simulink model "SMA_Wire_Sim"  (R2023b)
settings: Solver=VariableStepAuto  StartTime=0.0  StopTime=10  RelTol=1e-5
values from neighbouring files (symbols this model uses):
  Da = 75.0e9    (= 75000000000)    [Initialization.m]
  dens = 6450.0    (= 6450)    [Initialization.m]
  Dm = 28.0e9    (= 28000000000)    [Initialization.m]
  Dw = 0.00031    [Initialization.m]
  epsR = 0.05    [Initialization.m]
  epsR1 = 0.036    [Initialization.m]
  Length = 0.18    [Initialization.m]
  Lw1 = 0.18    [Initialization.m]
  Lw2 = 0.18    [Initialization.m]
  pa = 100*10^-8    (= 1e-06)    [Initialization.m]
  pm = 80*10^-8    (= 8e-07)    [Initialization.m]
  SectA = pi*(Diameter^2)/4    (= 7.54767635025e-08)    [Initialization.m]
  sigma0 = (disp_i*Ks)/SectA    (= 2649822.15346)    [Initialization.m]
  Tamb = 25    [Initialization.m]
  thetaT = 0    [Initialization.m]
libraries: nesl_utility x10, ee_lib x10, fl_lib x8, simulink_extras x4, simulink x3
(part 2 of 2)

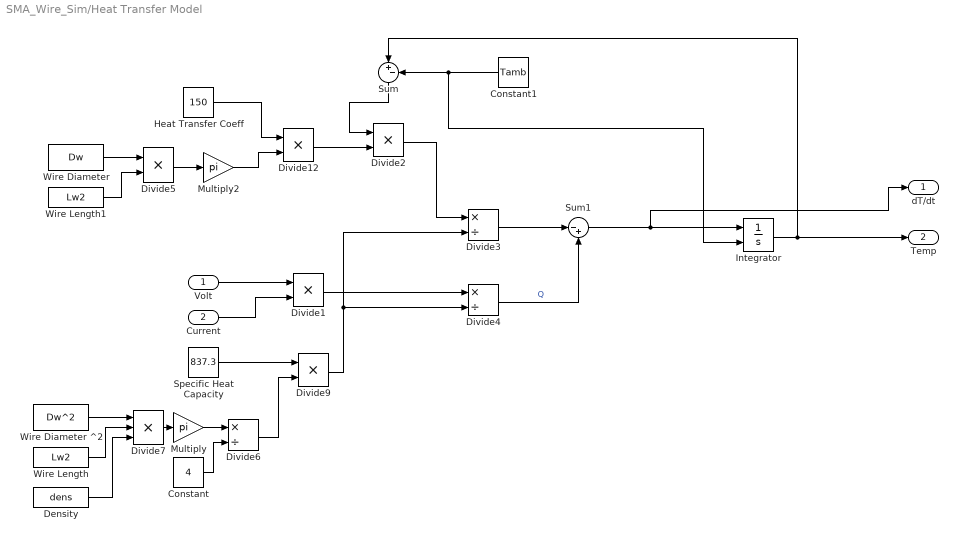
== system SMA_Wire_Sim/Heat Transfer Model ==
  Volt : Inport
  Current : Inport  Port=2
  Constant : Constant  Value=4
  Constant1 : Constant  Value=Tamb
  Density : Constant  Value=dens
  Divide{1..2,5,9,12} (5 alike) : Product  Inputs=**
  Divide3 : Product  Inputs=*/
  Divide4 : Product  Inputs=*/
  Divide6 : Product  Inputs=*/
  Divide7 : Product  Inputs=***
  Heat Transfer Coeff : Constant  Value=150
  Integrator : Integrator  InitialConditionSource=external  InitialCondition=25
  Multiply : Gain  Gain=pi
  Multiply2 : Gain  Gain=pi
  Specific Heat Capacity : Constant  Value=837.3
  Sum : Sum  Inputs=|+-
  Sum1 : Sum  Inputs=|-+
  Wire Diameter : Constant  Value=Dw
  Wire Diameter ^2 : Constant  Value=Dw^2
  Wire Length : Constant  Value=Lw2
  Wire Length1 : Constant  Value=Lw2
  dT/dt : Outport
  Temp : Outport  Port=2
  wires:
  Current/1 -> Divide1/2
  Volt/1 -> Divide1/1
  Constant1/1 -> Integrator/2, Sum/2
  Divide1/1 -> Divide4/1
  Wire Diameter ^2/1 -> Divide7/1
  Wire Length/1 -> Divide7/2
  Divide7/1 -> Multiply/1
  Divide3/1 -> Sum1/1
  Sum1/1 -> dT/dt/1, Integrator/1
  Divide4/1 -> Sum1/2  "Q"
  Density/1 -> Divide7/3
  Specific Heat Capacity/1 -> Divide9/1
  Multiply/1 -> Divide6/1
  Constant/1 -> Divide6/2
  Divide9/1 -> Divide3/2, Divide4/2
  Divide6/1 -> Divide9/2
  Sum/1 -> Divide2/1
  Divide2/1 -> Divide3/1
  Divide5/1 -> Multiply2/1
  Wire Length1/1 -> Divide5/2
  Wire Diameter/1 -> Divide5/1
  Multiply2/1 -> Divide12/2
  Heat Transfer Coeff/1 -> Divide12/1
  Divide12/1 -> Divide2/2
  Integrator/1 -> Sum/1, Temp/1

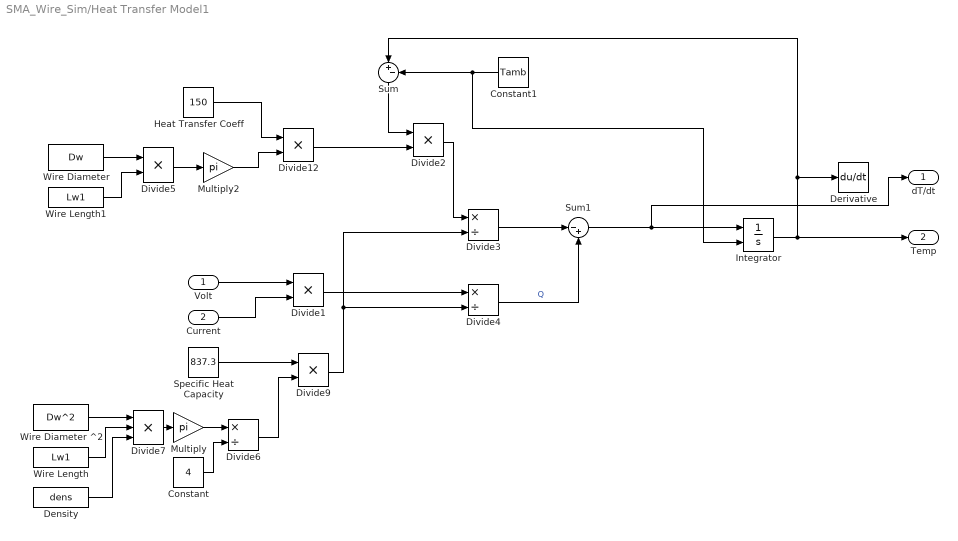
== system SMA_Wire_Sim/Heat Transfer Model1 ==
  Volt : Inport
  Current : Inport  Port=2
  Constant : Constant  Value=4
  Constant1 : Constant  Value=Tamb
  Density : Constant  Value=dens
  Derivative : Derivative
  Divide{1..2,5,9,12} (5 alike) : Product  Inputs=**
  Divide3 : Product  Inputs=*/
  Divide4 : Product  Inputs=*/
  Divide6 : Product  Inputs=*/
  Divide7 : Product  Inputs=***
  Heat Transfer Coeff : Constant  Value=150
  Integrator : Integrator  InitialConditionSource=external  InitialCondition=25
  Multiply : Gain  Gain=pi
  Multiply2 : Gain  Gain=pi
  Specific Heat Capacity : Constant  Value=837.3
  Sum : Sum  Inputs=|+-
  Sum1 : Sum  Inputs=|-+
  Wire Diameter : Constant  Value=Dw
  Wire Diameter ^2 : Constant  Value=Dw^2
  Wire Length : Constant  Value=Lw1
  Wire Length1 : Constant  Value=Lw1
  dT/dt : Outport
  Temp : Outport  Port=2
  wires:
  Current/1 -> Divide1/2
  Volt/1 -> Divide1/1
  Constant1/1 -> Sum/2, Integrator/2
  Divide1/1 -> Divide4/1
  Wire Diameter ^2/1 -> Divide7/1
  Wire Length/1 -> Divide7/2
  Divide7/1 -> Multiply/1
  Divide3/1 -> Sum1/1
  Sum1/1 -> dT/dt/1, Integrator/1
  Divide4/1 -> Sum1/2  "Q"
  Density/1 -> Divide7/3
  Specific Heat Capacity/1 -> Divide9/1
  Multiply/1 -> Divide6/1
  Constant/1 -> Divide6/2
  Divide9/1 -> Divide3/2, Divide4/2
  Divide6/1 -> Divide9/2
  Sum/1 -> Divide2/1
  Divide2/1 -> Divide3/1
  Divide5/1 -> Multiply2/1
  Wire Length1/1 -> Divide5/2
  Wire Diameter/1 -> Divide5/1
  Multiply2/1 -> Divide12/2
  Heat Transfer Coeff/1 -> Divide12/1
  Divide12/1 -> Divide2/2
  Integrator/1 -> Derivative/1, Sum/1, Temp/1

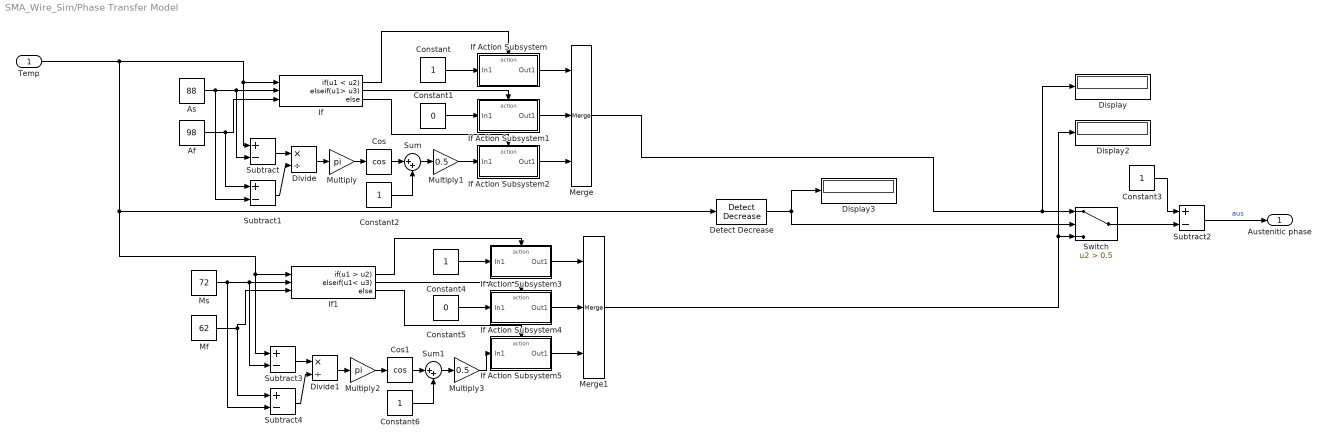
== system SMA_Wire_Sim/Phase Transfer Model ==
  Temp : Inport
  Af : Constant  Value=98
  As : Constant  Value=88
  Constant{,2..4,6} (5 alike) : Constant
  Constant1 : Constant  Value=0
  Constant5 : Constant  Value=0
  Cos : Trigonometry  Operator=cos
  Cos1 : Trigonometry  Operator=cos
  Detect Decrease : simulink/Logic and Bit Operations/Detect Decrease  vinit=0  OutDataTypeStr=uint8
  Display : Display
  Display2 : Display
  Display3 : Display
  Divide : Product  Inputs=*/
  Divide1 : Product  Inputs=*/
  If : If  NumInputs=3  IfExpression=u1 < u2  ElseIfExpressions=u1> u3
  If Action Subsystem : Subsystem  TreatAsAtomicUnit=on
  If Action Subsystem1 : Subsystem  TreatAsAtomicUnit=on
  If Action Subsystem2 : Subsystem  TreatAsAtomicUnit=on
  If Action Subsystem3 : Subsystem  TreatAsAtomicUnit=on
  If Action Subsystem4 : Subsystem  TreatAsAtomicUnit=on
  If Action Subsystem5 : Subsystem  TreatAsAtomicUnit=on
  If1 : If  NumInputs=3  IfExpression=u1 > u2  ElseIfExpressions=u1< u3
  Merge : Merge  Inputs=3
  Merge1 : Merge  Inputs=3
  Mf : Constant  Value=62
  Ms : Constant  Value=72
  Multiply : Gain  Gain=pi
  Multiply1 : Gain  Gain=0.5
  Multiply2 : Gain  Gain=pi
  Multiply3 : Gain  Gain=0.5
  Subtract{,1..4} (5 alike) : Sum  Inputs=+-
  Sum : Sum  Inputs=|++
  Sum1 : Sum  Inputs=|++
  Switch : Switch  Criteria=u2 > Threshold  Threshold=0.5  SaturateOnIntegerOverflow=off  InputSameDT=off
  "Austenitic phase " : Outport
  wires:
  As/1 -> Subtract1/2, Subtract/2, If/2
  Af/1 -> Subtract1/1, If/3
  If/1 -> If Action Subsystem/Action
  If/2 -> If Action Subsystem1/Action
  Constant/1 -> If Action Subsystem/1(In1)
  Constant1/1 -> If Action Subsystem1/1(In1)
  If/3 -> If Action Subsystem2/Action
  If Action Subsystem/1(Out1) -> Merge/1
  If Action Subsystem1/1(Out1) -> Merge/2
  If Action Subsystem2/1(Out1) -> Merge/3
  Subtract/1 -> Divide/1
  Subtract1/1 -> Divide/2
  Divide/1 -> Multiply/1
  Multiply/1 -> Cos/1
  Cos/1 -> Sum/1
  Constant2/1 -> Sum/2
  Sum/1 -> Multiply1/1
  Multiply1/1 -> If Action Subsystem2/1(In1)
  Constant3/1 -> Subtract2/1
  Divide1/1 -> Multiply2/1
  If Action Subsystem4/1(Out1) -> Merge1/2
  Multiply2/1 -> Cos1/1
  Mf/1 -> If1/3, Subtract4/1
  Cos1/1 -> Sum1/1
  Subtract3/1 -> Divide1/1
  Subtract4/1 -> Divide1/2
  Sum1/1 -> Multiply3/1
  Constant4/1 -> If Action Subsystem3/1(In1)
  If1/1 -> If Action Subsystem3/Action
  If1/3 -> If Action Subsystem5/Action
  If1/2 -> If Action Subsystem4/Action
  Constant5/1 -> If Action Subsystem4/1(In1)
  Ms/1 -> Subtract4/2, Subtract3/2, If1/2
  Constant6/1 -> Sum1/2
  Multiply3/1 -> If Action Subsystem5/1(In1)
  If Action Subsystem5/1(Out1) -> Merge1/3
  If Action Subsystem3/1(Out1) -> Merge1/1
  Temp/1 -> Detect Decrease/1, Subtract3/1, If1/1, Subtract/1, If/1
  Detect Decrease/1 -> Switch/2, Display3/1
  Merge1/1 -> Display2/1, Switch/3
  Merge/1 -> Display/1, Switch/1
  Switch/1 -> Subtract2/2
  Subtract2/1 -> "Austenitic phase "/1  "aus"

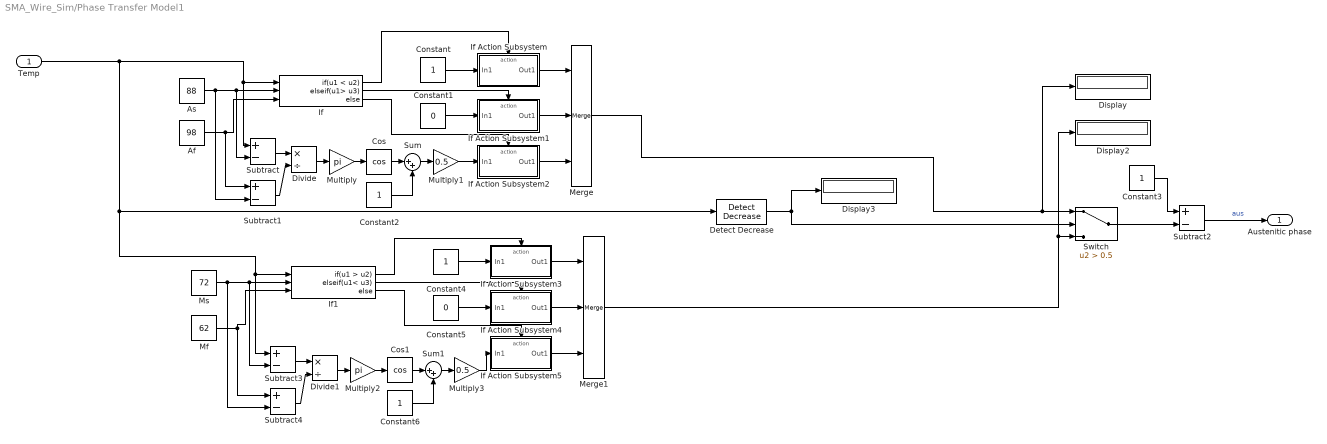
== system SMA_Wire_Sim/Phase Transfer Model1 ==
  Temp : Inport
  Af : Constant  Value=98
  As : Constant  Value=88
  Constant{,2..4,6} (5 alike) : Constant
  Constant1 : Constant  Value=0
  Constant5 : Constant  Value=0
  Cos : Trigonometry  Operator=cos
  Cos1 : Trigonometry  Operator=cos
  Detect Decrease : simulink/Logic and Bit Operations/Detect Decrease  vinit=0  OutDataTypeStr=uint8
  Display : Display
  Display2 : Display
  Display3 : Display
  Divide : Product  Inputs=*/
  Divide1 : Product  Inputs=*/
  If : If  NumInputs=3  IfExpression=u1 < u2  ElseIfExpressions=u1> u3
  If Action Subsystem : Subsystem  TreatAsAtomicUnit=on
  If Action Subsystem1 : Subsystem  TreatAsAtomicUnit=on
  If Action Subsystem2 : Subsystem  TreatAsAtomicUnit=on
  If Action Subsystem3 : Subsystem  TreatAsAtomicUnit=on
  If Action Subsystem4 : Subsystem  TreatAsAtomicUnit=on
  If Action Subsystem5 : Subsystem  TreatAsAtomicUnit=on
  If1 : If  NumInputs=3  IfExpression=u1 > u2  ElseIfExpressions=u1< u3
  Merge : Merge  Inputs=3
  Merge1 : Merge  Inputs=3
  Mf : Constant  Value=62
  Ms : Constant  Value=72
  Multiply : Gain  Gain=pi
  Multiply1 : Gain  Gain=0.5
  Multiply2 : Gain  Gain=pi
  Multiply3 : Gain  Gain=0.5
  Subtract{,1..4} (5 alike) : Sum  Inputs=+-
  Sum : Sum  Inputs=|++
  Sum1 : Sum  Inputs=|++
  Switch : Switch  Criteria=u2 > Threshold  Threshold=0.5  SaturateOnIntegerOverflow=off  InputSameDT=off
  "Austenitic phase " : Outport
  wires:
  As/1 -> Subtract1/2, Subtract/2, If/2
  Af/1 -> Subtract1/1, If/3
  If/1 -> If Action Subsystem/Action
  If/2 -> If Action Subsystem1/Action
  Constant/1 -> If Action Subsystem/1(In1)
  Constant1/1 -> If Action Subsystem1/1(In1)
  If/3 -> If Action Subsystem2/Action
  If Action Subsystem/1(Out1) -> Merge/1
  If Action Subsystem1/1(Out1) -> Merge/2
  If Action Subsystem2/1(Out1) -> Merge/3
  Subtract/1 -> Divide/1
  Subtract1/1 -> Divide/2
  Divide/1 -> Multiply/1
  Multiply/1 -> Cos/1
  Cos/1 -> Sum/1
  Constant2/1 -> Sum/2
  Sum/1 -> Multiply1/1
  Multiply1/1 -> If Action Subsystem2/1(In1)
  Constant3/1 -> Subtract2/1
  Divide1/1 -> Multiply2/1
  If Action Subsystem4/1(Out1) -> Merge1/2
  Multiply2/1 -> Cos1/1
  Mf/1 -> If1/3, Subtract4/1
  Cos1/1 -> Sum1/1
  Subtract3/1 -> Divide1/1
  Subtract4/1 -> Divide1/2
  Sum1/1 -> Multiply3/1
  Constant4/1 -> If Action Subsystem3/1(In1)
  If1/1 -> If Action Subsystem3/Action
  If1/3 -> If Action Subsystem5/Action
  If1/2 -> If Action Subsystem4/Action
  Constant5/1 -> If Action Subsystem4/1(In1)
  Ms/1 -> Subtract4/2, Subtract3/2, If1/2
  Constant6/1 -> Sum1/2
  Multiply3/1 -> If Action Subsystem5/1(In1)
  If Action Subsystem5/1(Out1) -> Merge1/3
  If Action Subsystem3/1(Out1) -> Merge1/1
  Temp/1 -> Detect Decrease/1, Subtract3/1, If1/1, Subtract/1, If/1
  Detect Decrease/1 -> Switch/2, Display3/1
  Merge1/1 -> Display2/1, Switch/3
  Merge/1 -> Display/1, Switch/1
  Switch/1 -> Subtract2/2
  Subtract2/1 -> "Austenitic phase "/1  "aus"

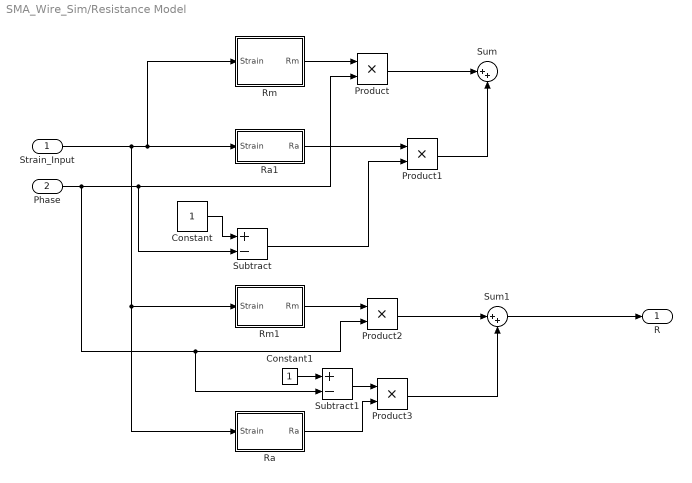
== system SMA_Wire_Sim/Resistance Model ==
  Strain_Input : Inport
  Phase : Inport  Port=2
  Constant : Constant
  Constant1 : Constant
  Product{,1..3} (4 alike) : Product
  Ra : Subsystem
  Ra1 : Subsystem
  Rm : Subsystem
  Rm1 : Subsystem
  Subtract : Sum  Inputs=+-
  Subtract1 : Sum  Inputs=+-
  Sum : Sum  Inputs=|++
  Sum1 : Sum  Inputs=|++
  R : Outport
  wires:
  Rm/1(Rm) -> Product/1
  Product/1 -> Sum/1
  Constant/1 -> Subtract/1
  Ra1/1(Ra) -> Product1/1
  Subtract/1 -> Product1/2
  Product1/1 -> Sum/2
  Strain_Input/1 -> Ra/1(Strain), Rm1/1(Strain), Ra1/1(Strain), Rm/1(Strain)
  Product3/1 -> Sum1/2
  Constant1/1 -> Subtract1/1
  Rm1/1(Rm) -> Product2/1
  Subtract1/1 -> Product3/1
  Product2/1 -> Sum1/1
  Ra/1(Ra) -> Product3/2
  Phase/1 -> Subtract1/2, Product2/2, Product/2, Subtract/2
  Sum1/1 -> R/1

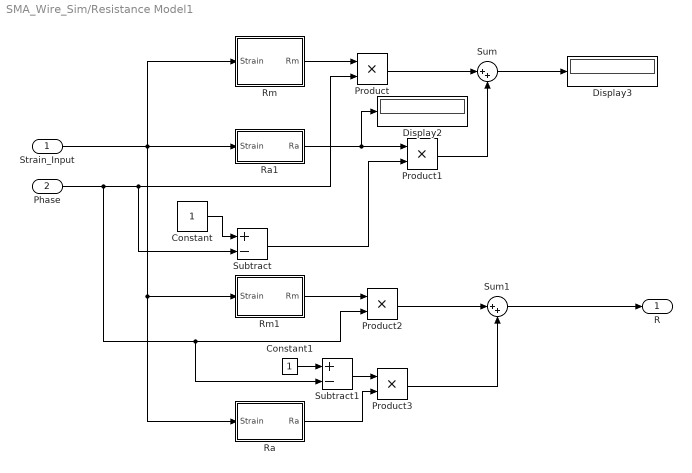
== system SMA_Wire_Sim/Resistance Model1 ==
  Strain_Input : Inport
  Phase : Inport  Port=2
  Constant : Constant
  Constant1 : Constant
  Display2 : Display
  Display3 : Display
  Product{,1..3} (4 alike) : Product
  Ra : Subsystem
  Ra1 : Subsystem
  Rm : Subsystem
  Rm1 : Subsystem
  Subtract : Sum  Inputs=+-
  Subtract1 : Sum  Inputs=+-
  Sum : Sum  Inputs=|++
  Sum1 : Sum  Inputs=|++
  R : Outport
  wires:
  Rm/1(Rm) -> Product/1
  Product/1 -> Sum/1
  Constant/1 -> Subtract/1
  Ra1/1(Ra) -> Display2/1, Product1/1
  Subtract/1 -> Product1/2
  Product1/1 -> Sum/2
  Sum/1 -> Display3/1
  Strain_Input/1 -> Rm/1(Strain), Ra/1(Strain), Rm1/1(Strain), Ra1/1(Strain)
  Product3/1 -> Sum1/2
  Constant1/1 -> Subtract1/1
  Rm1/1(Rm) -> Product2/1
  Subtract1/1 -> Product3/1
  Product2/1 -> Sum1/1
  Ra/1(Ra) -> Product3/2
  Phase/1 -> Subtract1/2, Product2/2, Product/2, Subtract/2
  Sum1/1 -> R/1

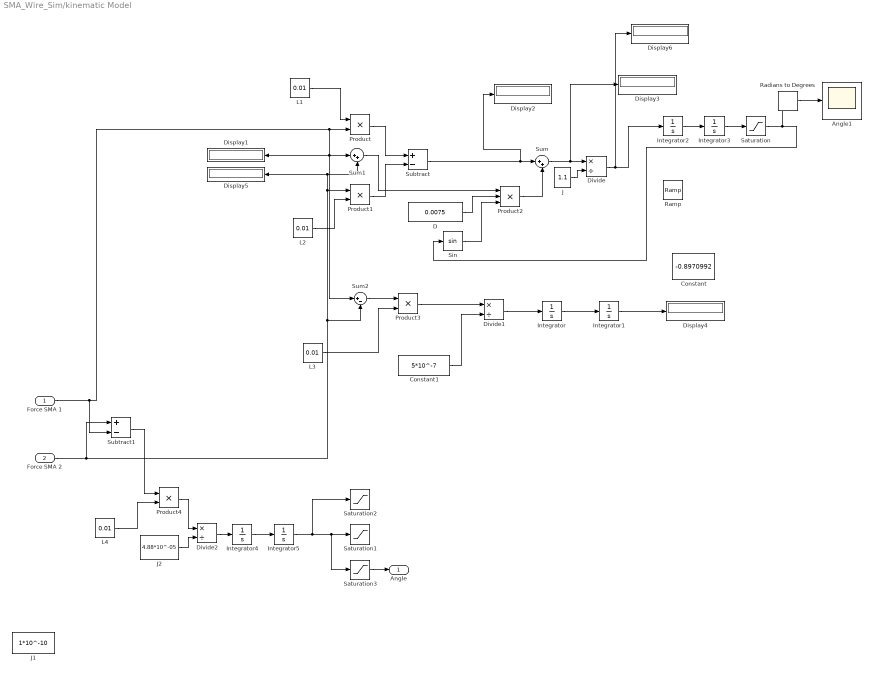
== system SMA_Wire_Sim/kinematic Model ==
  Force SMA 1 : Inport
  Force SMA 2 : Inport  Port=2
  Angle1 : Scope
  Constant : Constant  Value=-0.8970992
  Constant1 : Constant  Value=5*10^-7
  D : Constant  Value=0.0075
  Display{1..6} (6 alike) : Display
  Divide : Product  Inputs=*/
  Divide1 : Product  Inputs=*/
  Divide2 : Product  Inputs=*/
  Integrator{,1..5} (6 alike) : Integrator
  J : Constant  Value=1.1
  J1 : Constant  Value=1*10^-10
  J2 : Constant  Value=4.88*10^-05
  L{1..4} (4 alike) : Constant  Value=0.01
  Product{,1,3..4} (4 alike) : Product
  Product2 : Product  Inputs=3
  Radians to Degrees : simulink_extras/Transformations/Radians to Degrees
  Ramp : simulink/Sources/Ramp  slope=-0.25  start=0  InitialOutput=0
  Saturation : Saturate  UpperLimit=0.8970992  LowerLimit=-0.8970992
  Saturation1 : Saturate  UpperLimit=0.8970992  LowerLimit=-0.8970992
  Saturation2 : Saturate  UpperLimit=1.5708  LowerLimit=-1.5708
  Saturation3 : Saturate
  Sin : Trigonometry
  Subtract : Sum  Inputs=+-
  Subtract1 : Sum  Inputs=+-
  Sum : Sum  Inputs=|++
  Sum1 : Sum  Inputs=|++
  Sum2 : Sum  Inputs=|+-
  Angle : Outport
  wires:
  Force SMA 1/1 -> Subtract1/2, Sum2/1, Sum1/1, Display1/1, Product/2
  L1/1 -> Product/1
  L2/1 -> Product1/2
  Product/1 -> Subtract/1
  Product1/1 -> Subtract/2
  Force SMA 2/1 -> Subtract1/1, Sum1/2, Display5/1, Product1/1, Sum2/2
  D/1 -> Product2/2
  Sum1/1 -> Product2/1
  Sin/1 -> Product2/3
  Sum/1 -> Display3/1, Divide/1
  J/1 -> Divide/2
  Product2/1 -> Sum/2
  Integrator3/1 -> Saturation/1
  Divide/1 -> Integrator2/1, Display6/1
  Subtract/1 -> Display2/1, Sum/1
  Sum2/1 -> Product3/1
  L3/1 -> Product3/2
  Product3/1 -> Divide1/1
  Constant1/1 -> Divide1/2
  Divide1/1 -> Integrator/1
  Integrator/1 -> Integrator1/1
  Integrator1/1 -> Display4/1
  Integrator2/1 -> Integrator3/1
  Subtract1/1 -> Product4/1
  L4/1 -> Product4/2
  J2/1 -> Divide2/2
  Product4/1 -> Divide2/1
  Integrator4/1 -> Integrator5/1
  Divide2/1 -> Integrator4/1
  Integrator5/1 -> Saturation2/1, Saturation3/1, Saturation1/1
  Radians to Degrees/1 -> Angle1/1
  Saturation/1 -> Sin/1, Radians to Degrees/1
  Saturation3/1 -> Angle/1

== system SMA_Wire_Sim/Phase Transfer Model/If Action Subsystem ==
  In1 : Inport
  Action Port : ActionPort  ActionPortLabel=if(u1 < u2)
  Out1 : Outport
  wires:
  In1/1 -> Out1/1

== system SMA_Wire_Sim/Phase Transfer Model/If Action Subsystem1 ==
  In1 : Inport
  Action Port : ActionPort  ActionPortLabel=elseif(u1> u3)
  Out1 : Outport
  wires:
  In1/1 -> Out1/1

== system SMA_Wire_Sim/Phase Transfer Model/If Action Subsystem2 ==
  In1 : Inport
  Action Port : ActionPort  ActionPortLabel=else
  Out1 : Outport
  wires:
  In1/1 -> Out1/1

== system SMA_Wire_Sim/Phase Transfer Model/If Action Subsystem3 ==
  In1 : Inport
  Action Port : ActionPort  ActionPortLabel=if(u1 > u2)
  Out1 : Outport
  wires:
  In1/1 -> Out1/1

== system SMA_Wire_Sim/Phase Transfer Model/If Action Subsystem4 ==
  In1 : Inport
  Action Port : ActionPort  ActionPortLabel=elseif(u1< u3)
  Out1 : Outport
  wires:
  In1/1 -> Out1/1

== system SMA_Wire_Sim/Phase Transfer Model/If Action Subsystem5 ==
  In1 : Inport
  Action Port : ActionPort  ActionPortLabel=else
  Out1 : Outport
  wires:
  In1/1 -> Out1/1

== system SMA_Wire_Sim/Phase Transfer Model1/If Action Subsystem ==
  In1 : Inport
  Action Port : ActionPort  ActionPortLabel=if(u1 < u2)
  Out1 : Outport
  wires:
  In1/1 -> Out1/1

== system SMA_Wire_Sim/Phase Transfer Model1/If Action Subsystem1 ==
  In1 : Inport
  Action Port : ActionPort  ActionPortLabel=elseif(u1> u3)
  Out1 : Outport
  wires:
  In1/1 -> Out1/1

== system SMA_Wire_Sim/Phase Transfer Model1/If Action Subsystem2 ==
  In1 : Inport
  Action Port : ActionPort  ActionPortLabel=else
  Out1 : Outport
  wires:
  In1/1 -> Out1/1

== system SMA_Wire_Sim/Phase Transfer Model1/If Action Subsystem3 ==
  In1 : Inport
  Action Port : ActionPort  ActionPortLabel=if(u1 > u2)
  Out1 : Outport
  wires:
  In1/1 -> Out1/1

== system SMA_Wire_Sim/Phase Transfer Model1/If Action Subsystem4 ==
  In1 : Inport
  Action Port : ActionPort  ActionPortLabel=elseif(u1< u3)
  Out1 : Outport
  wires:
  In1/1 -> Out1/1

== system SMA_Wire_Sim/Phase Transfer Model1/If Action Subsystem5 ==
  In1 : Inport
  Action Port : ActionPort  ActionPortLabel=else
  Out1 : Outport
  wires:
  In1/1 -> Out1/1

== system SMA_Wire_Sim/Resistance Model/Ra ==
  Strain : Inport
  Divide : Product  Inputs=*/
  Product2 : Product
  Sum1 : Sum  Inputs=|++
  p_m : Constant  Value=pa
  p_m1 : Constant  Value=Length
  p_m2 : Constant  Value=SectA
  Ra : Outport
  wires:
  p_m1/1 -> Sum1/1
  Strain/1 -> Sum1/2
  p_m/1 -> Product2/1
  Sum1/1 -> Product2/2
  p_m2/1 -> Divide/2
  Product2/1 -> Divide/1
  Divide/1 -> Ra/1

== system SMA_Wire_Sim/Resistance Model/Ra1 ==
  Strain : Inport
  Constant : Constant
  Constant1 : Constant  Value=0.00031^2*pi
  Divide : Product  Inputs=*/
  Gain : Gain  Gain=4*.18
  Gain1 : Gain  Gain=2
  Product : Product
  Sum : Sum  Inputs=|++
  p_a : Constant  Value=100*10^-8
  Ra : Outport
  wires:
  Gain1/1 -> Sum/2
  Gain/1 -> Product/1
  p_a/1 -> Gain/1
  Constant1/1 -> Divide/2
  Product/1 -> Divide/1
  Constant/1 -> Sum/1
  Strain/1 -> Gain1/1
  Divide/1 -> Ra/1
  Sum/1 -> Product/2

== system SMA_Wire_Sim/Resistance Model/Rm ==
  Strain : Inport
  Constant : Constant
  Constant1 : Constant  Value=0.00031^2*pi
  Divide : Product  Inputs=*/
  Gain : Gain  Gain=4*.18
  Gain1 : Gain  Gain=2
  Product : Product
  Sum : Sum  Inputs=|++
  p_m : Constant  Value=80*10^-8
  Rm : Outport
  wires:
  Gain1/1 -> Sum/2
  Gain/1 -> Product/1
  p_m/1 -> Gain/1
  Constant1/1 -> Divide/2
  Product/1 -> Divide/1
  Constant/1 -> Sum/1
  Strain/1 -> Gain1/1
  Divide/1 -> Rm/1
  Sum/1 -> Product/2

== system SMA_Wire_Sim/Resistance Model/Rm1 ==
  Strain : Inport
  Divide : Product  Inputs=*/
  Product2 : Product
  Sum1 : Sum  Inputs=|++
  p_m : Constant  Value=pm
  p_m1 : Constant  Value=Length
  p_m2 : Constant  Value=SectA
  Rm : Outport
  wires:
  p_m1/1 -> Sum1/1
  Strain/1 -> Sum1/2
  p_m/1 -> Product2/1
  Sum1/1 -> Product2/2
  p_m2/1 -> Divide/2
  Product2/1 -> Divide/1
  Divide/1 -> Rm/1

== system SMA_Wire_Sim/Resistance Model1/Ra ==
  Strain : Inport
  Divide : Product  Inputs=*/
  Product2 : Product
  Sum1 : Sum  Inputs=|++
  p_m : Constant  Value=pa
  p_m1 : Constant  Value=Length
  p_m2 : Constant  Value=SectA
  Ra : Outport
  wires:
  p_m1/1 -> Sum1/1
  Strain/1 -> Sum1/2
  p_m/1 -> Product2/1
  Sum1/1 -> Product2/2
  p_m2/1 -> Divide/2
  Product2/1 -> Divide/1
  Divide/1 -> Ra/1

== system SMA_Wire_Sim/Resistance Model1/Ra1 ==
  Strain : Inport
  Constant : Constant
  Constant1 : Constant  Value=0.00031^2*pi
  Divide : Product  Inputs=*/
  Gain : Gain  Gain=4*.18
  Gain1 : Gain  Gain=2
  Product : Product
  Sum : Sum  Inputs=|++
  p_a : Constant  Value=100*10^-8
  Ra : Outport
  wires:
  Gain1/1 -> Sum/2
  Gain/1 -> Product/1
  p_a/1 -> Gain/1
  Constant1/1 -> Divide/2
  Product/1 -> Divide/1
  Constant/1 -> Sum/1
  Strain/1 -> Gain1/1
  Divide/1 -> Ra/1
  Sum/1 -> Product/2

== system SMA_Wire_Sim/Resistance Model1/Rm ==
  Strain : Inport
  Constant : Constant
  Constant1 : Constant  Value=0.00031^2*pi
  Divide : Product  Inputs=*/
  Gain : Gain  Gain=4*.18
  Gain1 : Gain  Gain=2
  Product : Product
  Sum : Sum  Inputs=|++
  p_m : Constant  Value=80*10^-8
  Rm : Outport
  wires:
  Gain1/1 -> Sum/2
  Gain/1 -> Product/1
  p_m/1 -> Gain/1
  Constant1/1 -> Divide/2
  Product/1 -> Divide/1
  Constant/1 -> Sum/1
  Strain/1 -> Gain1/1
  Divide/1 -> Rm/1
  Sum/1 -> Product/2

== system SMA_Wire_Sim/Resistance Model1/Rm1 ==
  Strain : Inport
  Divide : Product  Inputs=*/
  Product2 : Product
  Sum1 : Sum  Inputs=|++
  p_m : Constant  Value=pm
  p_m1 : Constant  Value=Length
  p_m2 : Constant  Value=SectA
  Rm : Outport
  wires:
  p_m1/1 -> Sum1/1
  Strain/1 -> Sum1/2
  p_m/1 -> Product2/1
  Sum1/1 -> Product2/2
  p_m2/1 -> Divide/2
  Product2/1 -> Divide/1
  Divide/1 -> Rm/1
